simulink model "one_factor"  (Simulink 7.0)
settings: Solver=ode4  StartTime=0.0  StopTime=10.0  FixedStep=0.01  RelTol=1e-3
undefined symbols (not defined in the file or in its folder): slcm
libraries: simulink x2
settings Model: Creator=xux  LastModifiedBy=jza
settings DebuggingCC: SaveWithParameterizedLinksMsg=none
settings GRTTargetCC: TargetFcnLib=ansi_tfl_tmw.mat

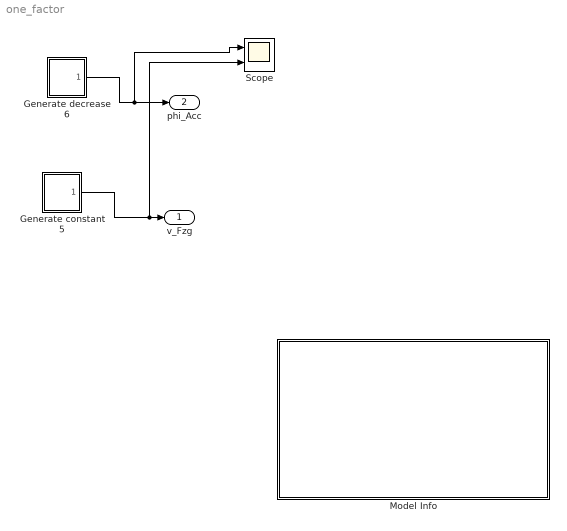
== system one_factor ==
  Generate constant 5 : Subsystem
  Generate decrease 6 : Subsystem
  Model Info : Subsystem  LoadFcn=slcm LoadBlock;  InitFcn=slcm('UpdateAllCMBlocksInThisModelInit')  mask(CMBlock){InitialSaveTempField=, InitialBlockCM=None, BlockCM=None, Frame=on, SaveTempField=, DisplayStringWithTags=|, MaskDisplayString=jza - 14.05.08\n\nThis is a prototypical relaization of the combination strategy - one factor at a time, which is nt implemented in the transformer, but it works here. \n\nFor the TDG unit, test control algorithm would have to be adjusted. \nprobably also sequencing of data would have to be adjusted., HorizontalTextAlignment=Center, LeftAlignmentValue=0.5, SourceBlockDiagram=one_factor, TagMaxNumber=20, CMTag1=, CMTag2=, CMTag3=, CMTag4=, CMTag5=, CMTag6=, CMTag7=, CMTag8=, CMTag9=, CMTag10=, CMTag11=, CMTag12=, CMTag13=, CMTag14=, CMTag15=, CMTag16=, CMTag17=, CMTag18=, CMTag19=, CMTag20=}
      mask DisplayStringWithTags=|
      | jza - 14.05.08
      |
      | This is a prototypical relaization of the combination strategy - one factor at a time, which is nt implemented in the transformer, but it works here.
      |
      | For the TDG unit, test control algorithm would have to be adjusted.
      | probably also sequencing of data would have to be adjusted.
      mask help: This block allows revision control information to be displayed within the model.
      settings: CopyFcn=slcm CopyBlock;  DeleteFcn=slcm Cancel;  PostSaveFcn=slcm('UpdateAllCMBlocksInThisModel')  NameChangeFcn=slcm Rename;  OpenFcn=slcm
      mask Display: text(str2num(LeftAlignmentValue), 0.5, MaskDisplayString, 'HorizontalAlignment', HorizontalTextAlignment)
  Scope : Scope  NumInputPorts=2
      settings: YMin=-5~-5  YMax=5~5
  v_Fzg : Outport  OutDataType=sfix(16)  OutScaling=2^0
  phi_Acc : Outport  Port=2  OutDataType=sfix(16)  OutScaling=2^0
  wires:
  Generate constant 5/1(v_Fzg) -> v_Fzg/1, Scope/2
  Generate decrease 6/1(phi_Acc) -> phi_Acc/1, Scope/1

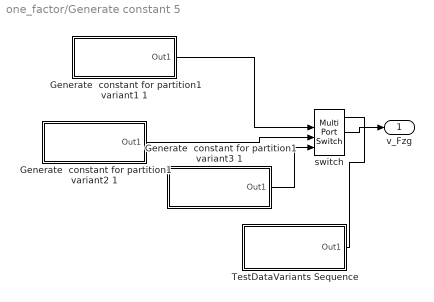
== system one_factor/Generate constant 5 ==
  Generate  constant for partition1 variant1 1 : Subsystem  mask(Feature generation){X0=-10, T=2}
      mask prompts: X0 "Constant value:"; T "Duration"
      mask help: Output a decreasing ramp signal limited from bottom and top, starting at the specified time.
      mask Display: plot([1:2],[4,4])
  Generate  constant for partition1 variant2 1 : Subsystem  mask(Feature generation){X0=70, T=2}
      mask prompts: X0 "Constant value:"; T "Duration"
      mask help: Output a decreasing ramp signal limited from bottom and top, starting at the specified time.
      mask Display: plot([1:2],[4,4])
  Generate  constant for partition1 variant3 1 : Subsystem  mask(Feature generation){X0=0, T=20}
      mask prompts: X0 "Constant value:"; T "Duration"
      mask help: Output a decreasing ramp signal limited from bottom and top, starting at the specified time.
      mask Display: plot([1:2],[4,4])
  TestDataVariants Sequence : Subsystem
  switch : MultiPortSwitch  Inputs=3
  v_Fzg : Outport  OutDataType=sfix(16)  OutScaling=2^0
  wires:
  switch/1 -> v_Fzg/1
  Generate  constant for partition1 variant2 1/1(Out1) -> switch/3
  Generate  constant for partition1 variant1 1/1(Out1) -> switch/2
  Generate  constant for partition1 variant3 1/1(Out1) -> switch/4
  TestDataVariants Sequence/1(Out1) -> switch/1

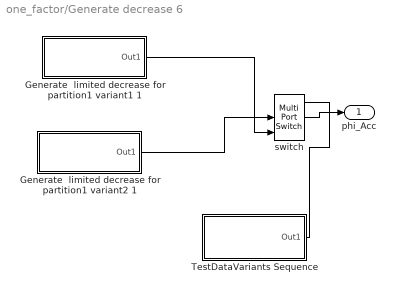
== system one_factor/Generate decrease 6 ==
  Generate  limited decrease for partition1 variant1 1 : Subsystem  mask(Feature generation){X0=28, XF=2, T=2}
      mask prompts: X0 "Initial output:"; XF "Final output:"; T "Duration"
      mask help: Output a decreasing ramp signal limited from bottom and top, starting at the specified time.
      mask Display:
      | plot([1:10],[4,4,4,4,4,1,1,1,1,1])
      | plot([1:10],[4,4,4,1,1,1,1,1,1,1])
      | plot([1:10],[4,1,1,1,1,1,1,1,1,1])
      | plot([1:10],[4,4,4,4,4,1,1,1,1,1])
      | plot([1:10],[4,4,4,4,4,4,4,1,1,1])
      | plot([1:10],[4,4,4,4,4,4,4,4,4,1])
      | plot([1:10],[4,4,4,4,4,4,4,4,4,4])
      | color('white');
      | plot([1:10],[1,1,1,1,1,1,1,1,1,1])
      | color('black');
      | plot([1,1.5],[1,1])
      | plot([2.5,3.5],[1,1])
      | plot([4.5,5.5],[1,1])
      | plot([6.5,7.5],[1,1])
      | plot([8.5,9.5],[1,1])
      | color('white');
      | plot([1,1.5],[4,4])
      | plot([2.5,3.5],[4,4])
      | plot([4.5,5.5],[4,4])
      | plot([6.5,7.5],[4,4])
      | plot([8.5,9.5],[4,4])
  Generate  limited decrease for partition1 variant2 1 : Subsystem  mask(Feature generation){X0=100, XF=92, T=2}
      mask prompts: X0 "Initial output:"; XF "Final output:"; T "Duration"
      mask help: Output a decreasing ramp signal limited from bottom and top, starting at the specified time.
      mask Display:
      | plot([1:10],[4,4,4,4,4,1,1,1,1,1])
      | plot([1:10],[4,4,4,1,1,1,1,1,1,1])
      | plot([1:10],[4,1,1,1,1,1,1,1,1,1])
      | plot([1:10],[4,4,4,4,4,1,1,1,1,1])
      | plot([1:10],[4,4,4,4,4,4,4,1,1,1])
      | plot([1:10],[4,4,4,4,4,4,4,4,4,1])
      | plot([1:10],[4,4,4,4,4,4,4,4,4,4])
      | color('white');
      | plot([1:10],[1,1,1,1,1,1,1,1,1,1])
      | color('black');
      | plot([1,1.5],[1,1])
      | plot([2.5,3.5],[1,1])
      | plot([4.5,5.5],[1,1])
      | plot([6.5,7.5],[1,1])
      | plot([8.5,9.5],[1,1])
      | color('white');
      | plot([1,1.5],[4,4])
      | plot([2.5,3.5],[4,4])
      | plot([4.5,5.5],[4,4])
      | plot([6.5,7.5],[4,4])
      | plot([8.5,9.5],[4,4])
  TestDataVariants Sequence : Subsystem
  switch : MultiPortSwitch  Inputs=2
  phi_Acc : Outport  OutDataType=sfix(16)  OutScaling=2^0
  wires:
  switch/1 -> phi_Acc/1
  TestDataVariants Sequence/1(Out1) -> switch/1
  Generate  limited decrease for partition1 variant2 1/1(Out1) -> switch/2
  Generate  limited decrease for partition1 variant1 1/1(Out1) -> switch/3

== system one_factor/Model Info ==
  EmptySubsystem : Subsystem

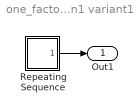
== system one_factor/Generate constant 5/Generate  constant for partition1 variant1 1 ==
  Repeating Sequence : Subsystem  mask(Repeating table){rep_seq_t=[0 T], rep_seq_y=[X0 X0]}
      mask prompts: rep_seq_t "Time values:"; rep_seq_y "Output values:"
      mask help: Output a repeating sequence of numbers specified in a table of time-value pairs. Values of time should be monotonically increasing.
      mask init:
      | if (length(rep_seq_t) ~= length(rep_seq_y)),
      |   error('Length of time vector and output vector must be the same.')
      | end
      | dbl_rep_seq_t = double(rep_seq_t);
      | dbl_rep_seq_y = double(rep_seq_y);
      | period = max(dbl_rep_seq_t) - min(dbl_rep_seq_t);
      | s = round(length(dbl_rep_seq_t)/50);
      | if s > 0
      |   pts = [1:s:length(dbl_rep_seq_t)];
      |   L   = length(pts);
      | else
      |   L   = length(dbl_rep_seq_t);
      |   pts = [1:L];
      | end
      | 
      | disp_seq_t = reshape(dbl_rep_seq_t(pts),L,1);
      | disp_seq_y = reshape(dbl_rep_seq_y(pts),L,1);
      | disp_period = max(disp_seq_t) - min(disp_seq_t);
      | 
      | disp_seq_t  = repmat(disp_seq_t,1,3) + (ones(L,1)*(disp_period*[0,1,2]));
      | disp_seq_t = [ disp_seq_t(:); disp_seq_t(end) ];
      | disp_seq_y = repmat(disp_seq_y,1,3);
      | disp_seq_y = [ disp_seq_y(:); disp_seq_y(1) ];
      mask Help: Repeats cycle given in table. Time values should be monotonically increasing.
      mask Display: plot( disp_seq_t, disp_seq_y )
  Out1 : Outport  OutDataType=sfix(16)  OutScaling=2^0
  wires:
  Repeating Sequence/1(Out1) -> Out1/1

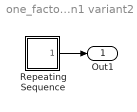
== system one_factor/Generate constant 5/Generate  constant for partition1 variant2 1 ==
  Repeating Sequence : Subsystem  mask(Repeating table){rep_seq_t=[0 T], rep_seq_y=[X0 X0]}
      mask prompts: rep_seq_t "Time values:"; rep_seq_y "Output values:"
      mask help: Output a repeating sequence of numbers specified in a table of time-value pairs. Values of time should be monotonically increasing.
      mask init: same as one_factor/Generate constant 5/Generate  constant for partition1 variant1 1/Repeating Sequence
      mask Help: Repeats cycle given in table. Time values should be monotonically increasing.
      mask Display: plot( disp_seq_t, disp_seq_y )
  Out1 : Outport  OutDataType=sfix(16)  OutScaling=2^0
  wires:
  Repeating Sequence/1(Out1) -> Out1/1

== system one_factor/Generate constant 5/Generate  constant for partition1 variant3 1 ==
  Repeating Sequence : Subsystem  mask(Repeating table){rep_seq_t=[0 T], rep_seq_y=[X0 X0]}
      mask prompts: rep_seq_t "Time values:"; rep_seq_y "Output values:"
      mask help: Output a repeating sequence of numbers specified in a table of time-value pairs. Values of time should be monotonically increasing.
      mask init: same as one_factor/Generate constant 5/Generate  constant for partition1 variant1 1/Repeating Sequence
      mask Help: Repeats cycle given in table. Time values should be monotonically increasing.
      mask Display: plot( disp_seq_t, disp_seq_y )
  Out1 : Outport  OutDataType=sfix(16)  OutScaling=2^0
  wires:
  Repeating Sequence/1(Out1) -> Out1/1

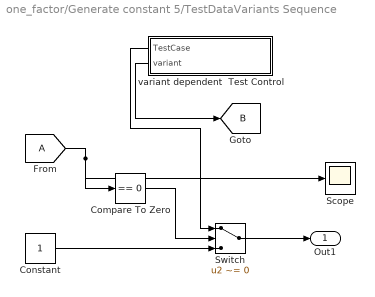
== system one_factor/Generate constant 5/TestDataVariants Sequence ==
  Compare To Zero : simulink/Logic and Bit Operations/Compare To Zero  SystemSampleTime=-1  relop===  LogicOutDataTypeMode=uint8  ZeroCross=off
  Constant : Constant  OutDataType=sfix(16)  OutScaling=2^0
  Scope : Scope
      settings: SaveName=ScopeData2
  Switch : Switch  Criteria=u2 ~= 0  Threshold=1
  variant dependent  Test Control : Stateflow chart  Orientation=left  AncestorBlock=|
      | MIL_Test/Test Control/Test Control Architecture/variant dependent 
      | Test Control/variant dependent 
      | Test Control
  Out1 : Outport  OutDataType=sfix(16)  OutScaling=2^0
  tag scope: B=global
  wires:
  Constant/1 -> Switch/3
  Switch/1 -> Out1/1
  variant dependent  Test Control/1(TestCase) -> Switch/1
  [A] -> Compare To Zero/1, Scope/1
  Compare To Zero/1 -> Switch/2
  variant dependent  Test Control/2(variant) -> [B]

== system one_factor/Generate decrease 6/Generate  limited decrease for partition1 variant1 1 ==
  Repeating Sequence : Subsystem  mask(Repeating table){rep_seq_t=[0 T], rep_seq_y=[X0 XF]}
      mask prompts: rep_seq_t "Time values:"; rep_seq_y "Output values:"
      mask help: Output a repeating sequence of numbers specified in a table of time-value pairs. Values of time should be monotonically increasing.
      mask init: same as one_factor/Generate constant 5/Generate  constant for partition1 variant1 1/Repeating Sequence
      mask Help: Repeats cycle given in table. Time values should be monotonically increasing.
      mask Display: plot( disp_seq_t, disp_seq_y )
  Out1 : Outport  OutDataType=sfix(16)  OutScaling=2^0
  wires:
  Repeating Sequence/1(Out1) -> Out1/1

== system one_factor/Generate decrease 6/Generate  limited decrease for partition1 variant2 1 ==
  Repeating Sequence : Subsystem  mask(Repeating table){rep_seq_t=[0 T], rep_seq_y=[X0 XF]}
      mask prompts: rep_seq_t "Time values:"; rep_seq_y "Output values:"
      mask help: Output a repeating sequence of numbers specified in a table of time-value pairs. Values of time should be monotonically increasing.
      mask init: same as one_factor/Generate constant 5/Generate  constant for partition1 variant1 1/Repeating Sequence
      mask Help: Repeats cycle given in table. Time values should be monotonically increasing.
      mask Display: plot( disp_seq_t, disp_seq_y )
  Out1 : Outport  OutDataType=sfix(16)  OutScaling=2^0
  wires:
  Repeating Sequence/1(Out1) -> Out1/1

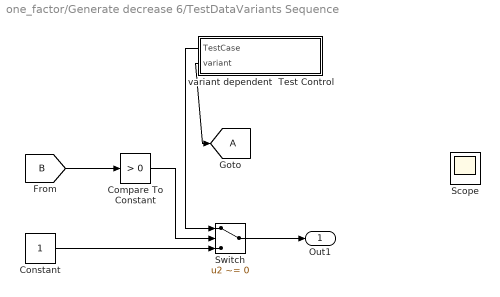
== system one_factor/Generate decrease 6/TestDataVariants Sequence ==
  Compare To Constant : simulink/Logic and Bit Operations/Compare To Constant  SystemSampleTime=-1  relop=>  const=0  LogicOutDataTypeMode=uint8  ZeroCross=off
  Constant : Constant  OutDataType=sfix(16)  OutScaling=2^0
  Scope : Scope
  Switch : Switch  Criteria=u2 ~= 0  Threshold=3
  variant dependent  Test Control : Stateflow chart  Orientation=left  AncestorBlock=|
      | MIL_Test/Test Control/Test Control Architecture/variant dependent 
      | Test Control/variant dependent 
      | Test Control
  Out1 : Outport  OutDataType=sfix(16)  OutScaling=2^0
  tag scope: A=global
  wires:
  Constant/1 -> Switch/3
  Switch/1 -> Out1/1
  [B] -> Compare To Constant/1
  variant dependent  Test Control/2(variant) -> [A]
  variant dependent  Test Control/1(TestCase) -> Switch/1
  Compare To Constant/1 -> Switch/2

== system one_factor/Model Info/EmptySubsystem ==

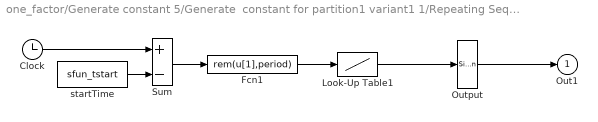
== system one_factor/Generate constant 5/Generate  constant for partition1 variant1 1/Repeating Sequence ==
  Clock : Clock
      settings: Decimation=10
  Fcn1 : Fcn  Expr=rem(u[1],period)
  Look-Up Table1 : Lookup  InputValues=rep_seq_t - min(rep_seq_t)  Table=rep_seq_y  OutDataType=sfix(16)  OutScaling=2^0  SaturateOnIntegerOverflow=on
  Output : SignalConversion  ConversionOutput=Contiguous copy
  Sum : Sum  Inputs=+-  OutDataType=sfix(16)  OutScaling=2^0  SaturateOnIntegerOverflow=on  InputSameDT=on
  startTime : S-Function  FunctionName=sfun_tstart
  Out1 : Outport  OutDataType=sfix(16)  OutScaling=2^0
  wires:
  Output/1 -> Out1/1
  Look-Up Table1/1 -> Output/1
  startTime/1 -> Sum/2
  Clock/1 -> Sum/1
  Sum/1 -> Fcn1/1
  Fcn1/1 -> Look-Up Table1/1

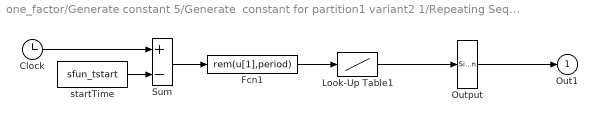
== system one_factor/Generate constant 5/Generate  constant for partition1 variant2 1/Repeating Sequence ==
  Clock : Clock
      settings: Decimation=10
  Fcn1 : Fcn  Expr=rem(u[1],period)
  Look-Up Table1 : Lookup  InputValues=rep_seq_t - min(rep_seq_t)  Table=rep_seq_y  OutDataType=sfix(16)  OutScaling=2^0  SaturateOnIntegerOverflow=on
  Output : SignalConversion  ConversionOutput=Contiguous copy
  Sum : Sum  Inputs=+-  OutDataType=sfix(16)  OutScaling=2^0  SaturateOnIntegerOverflow=on  InputSameDT=on
  startTime : S-Function  FunctionName=sfun_tstart
  Out1 : Outport  OutDataType=sfix(16)  OutScaling=2^0
  wires:
  Output/1 -> Out1/1
  Look-Up Table1/1 -> Output/1
  startTime/1 -> Sum/2
  Clock/1 -> Sum/1
  Sum/1 -> Fcn1/1
  Fcn1/1 -> Look-Up Table1/1

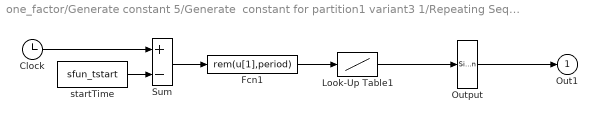
== system one_factor/Generate constant 5/Generate  constant for partition1 variant3 1/Repeating Sequence ==
  Clock : Clock
      settings: Decimation=10
  Fcn1 : Fcn  Expr=rem(u[1],period)
  Look-Up Table1 : Lookup  InputValues=rep_seq_t - min(rep_seq_t)  Table=rep_seq_y  OutDataType=sfix(16)  OutScaling=2^0  SaturateOnIntegerOverflow=on
  Output : SignalConversion  ConversionOutput=Contiguous copy
  Sum : Sum  Inputs=+-  OutDataType=sfix(16)  OutScaling=2^0  SaturateOnIntegerOverflow=on  InputSameDT=on
  startTime : S-Function  FunctionName=sfun_tstart
  Out1 : Outport  OutDataType=sfix(16)  OutScaling=2^0
  wires:
  Output/1 -> Out1/1
  Look-Up Table1/1 -> Output/1
  startTime/1 -> Sum/2
  Clock/1 -> Sum/1
  Sum/1 -> Fcn1/1
  Fcn1/1 -> Look-Up Table1/1

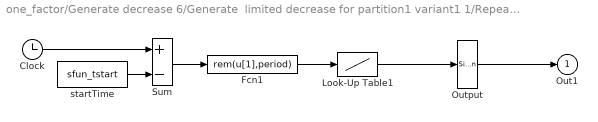
== system one_factor/Generate decrease 6/Generate  limited decrease for partition1 variant1 1/Repeating Sequence ==
  Clock : Clock
      settings: Decimation=10
  Fcn1 : Fcn  Expr=rem(u[1],period)
  Look-Up Table1 : Lookup  InputValues=rep_seq_t - min(rep_seq_t)  Table=rep_seq_y  OutDataType=sfix(16)  OutScaling=2^0  SaturateOnIntegerOverflow=on
  Output : SignalConversion  ConversionOutput=Contiguous copy
  Sum : Sum  Inputs=+-  OutDataType=sfix(16)  OutScaling=2^0  SaturateOnIntegerOverflow=on  InputSameDT=on
  startTime : S-Function  FunctionName=sfun_tstart
  Out1 : Outport  OutDataType=sfix(16)  OutScaling=2^0
  wires:
  Fcn1/1 -> Look-Up Table1/1
  Sum/1 -> Fcn1/1
  Clock/1 -> Sum/1
  startTime/1 -> Sum/2
  Look-Up Table1/1 -> Output/1
  Output/1 -> Out1/1

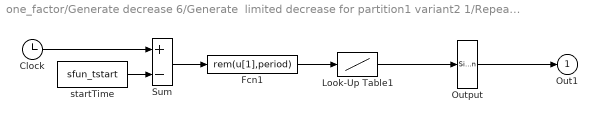
== system one_factor/Generate decrease 6/Generate  limited decrease for partition1 variant2 1/Repeating Sequence ==
  Clock : Clock
      settings: Decimation=10
  Fcn1 : Fcn  Expr=rem(u[1],period)
  Look-Up Table1 : Lookup  InputValues=rep_seq_t - min(rep_seq_t)  Table=rep_seq_y  OutDataType=sfix(16)  OutScaling=2^0  SaturateOnIntegerOverflow=on
  Output : SignalConversion  ConversionOutput=Contiguous copy
  Sum : Sum  Inputs=+-  OutDataType=sfix(16)  OutScaling=2^0  SaturateOnIntegerOverflow=on  InputSameDT=on
  startTime : S-Function  FunctionName=sfun_tstart
  Out1 : Outport  OutDataType=sfix(16)  OutScaling=2^0
  wires:
  Fcn1/1 -> Look-Up Table1/1
  Sum/1 -> Fcn1/1
  Clock/1 -> Sum/1
  startTime/1 -> Sum/2
  Look-Up Table1/1 -> Output/1
  Output/1 -> Out1/1

== stateflow chart Generate constant 5/TestDataVariants Sequence/variant dependent Test Control ==
  state TestCase1
    entry: TestCase = 1;
  state TestCase2
    entry: TestCase = 2;
  state Stop
  state TestCase3
    entry: TestCase = 3;
  (default) -> TestCase1 : {variant=0;}
  (junction 7) -> TestCase1 : {variant=variant+1;}
  TestCase2 -> TestCase3 : after(200, tick)
  TestCase1 -> TestCase2 : after(200, tick)
  Stop -> (junction 7)
  TestCase3 -> Stop : after(200, tick)
  data: TestCase output double; variant output double

== stateflow chart Generate decrease 6/TestDataVariants Sequence/variant dependent Test Control ==
  state TestCase1
    entry: TestCase = 1;
  state TestCase2
    entry: TestCase = 2;
  state Stop
  state TestCase0
    entry: TestCase = 1;
  (default) -> TestCase0 : {variant=0;}
  (junction 22) -> TestCase1
  TestCase2 -> Stop : after(200, tick)
  TestCase1 -> TestCase2 : after(200, tick)
  Stop -> (junction 22) : {variant=variant+1;}
  TestCase0 -> TestCase1 : after(400, tick)
  data: TestCase output double; variant output double
